simulink model "ejemplo_mimo"  (R2018a)
settings: Solver=VariableStepAuto  StartTime=0.0  StopTime=10  RelTol=1e-3
InitFcn:
  | ej_mimo2
values from neighbouring files (symbols this model uses):
  ki = kt(1,3)    [control_nolineal_linealizacion_entrada_estado.m]    (also in e_mimo.m; ej_mimo.m = kt(:,2+1:end); ej_mimo2.m = kt(:,2+1:end); ejemplo_2.m)
  kp = kt(1,1:2)    [control_nolineal_linealizacion_entrada_estado.m]    (also in e_mimo.m; ej_mimo.m = kt(:,1:2); ej_mimo2.m = kt(:,1:2); ejemplo_2.m)
libraries: simulink x2
settings Model: Creator=carma  LastModifiedBy=carma

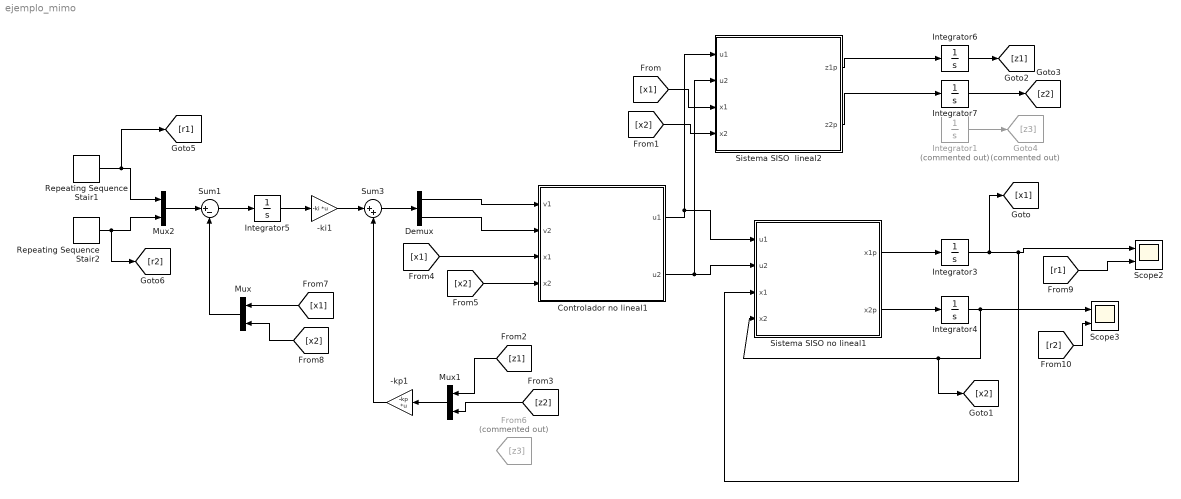
== system ejemplo_mimo ==
  -ki1 : Gain  Gain=-ki  Multiplication=Matrix(K*u) (u vector)
  -kp1 : Gain  Gain=-kp  Multiplication=Matrix(K*u) (u vector)
  Controlador no lineal1 : MATLAB Function  TreatAsAtomicUnit=on
  Demux : Demux  Outputs=2
  From6 : From  Commented=on  GotoTag=z3
  Goto4 : Goto  Commented=on  GotoTag=z3
  Integrator1 : Integrator  Commented=on
  Integrator{3..7} (5 alike) : Integrator
  Mux : Mux  Inputs=2
  Mux1 : Mux  Inputs=2
  Mux2 : Mux  Inputs=2
  Repeating Sequence Stair1 : simulink/Sources/Repeating Sequence Stair  OutValues=[0.5 0.4 -0.2 0.1 0.3].'  tsamp=2  OutMin=[]  OutMax=[]  OutDataTypeStr=double  OutputDataTypeScalingMode=double  OutDataType=fixdt(0,8)  ConRadixGroup=Best Precision: Vector-wise  OutScaling=2^-12
  Repeating Sequence Stair2 : simulink/Sources/Repeating Sequence Stair  OutValues=[-0.5 -0.4 0.2 -0.1 -0.3].'  tsamp=1.5  OutMin=[]  OutMax=[]  OutDataTypeStr=double  OutputDataTypeScalingMode=double  OutDataType=fixdt(0,8)  ConRadixGroup=Best Precision: Vector-wise  OutScaling=2^-12
  Scope2 : Scope  NumInputPorts=2
  Scope3 : Scope  NumInputPorts=2
  Sistema SISO  lineal2 : MATLAB Function  TreatAsAtomicUnit=on
  Sistema SISO no lineal1 : MATLAB Function  TreatAsAtomicUnit=on
  Sum1 : Sum  Inputs=|+-
  Sum3 : Sum  Inputs=|++
  wires:
  Sistema SISO  lineal2/1(z1p) -> Integrator6/1
  Sistema SISO no lineal1/2(x2p) -> Integrator4/1
  Sum1/1 -> Integrator5/1
  Controlador no lineal1/1(u1) -> Sistema SISO no lineal1/1(u1), Sistema SISO  lineal2/1(u1)
  Sistema SISO no lineal1/1(x1p) -> Integrator3/1
  Integrator4/1 -> [x2], Sistema SISO no lineal1/4(x2), Scope3/1
  Mux1/1 -> -kp1/1
  Integrator5/1 -> -ki1/1
  Sistema SISO  lineal2/2(z2p) -> Integrator7/1
  -ki1/1 -> Sum3/1
  -kp1/1 -> Sum3/2
  Integrator3/1 -> [x1], Scope2/1, Sistema SISO no lineal1/3(x1)
  [x1] -> Sistema SISO  lineal2/3(x1)
  [x2] -> Sistema SISO  lineal2/4(x2)
  Integrator6/1 -> [z1]
  Integrator7/1 -> [z2]
  [z1] -> Mux1/1
  [z2] -> Mux1/2
  Integrator1/1 -> Goto4/1
  Mux2/1 -> Sum1/1
  Repeating Sequence Stair1/1 -> [r1], Mux2/1
  Repeating Sequence Stair2/1 -> [r2], Mux2/2
  [x1] -> Mux/1
  [x2] -> Mux/2
  Mux/1 -> Sum1/2
  [r1] -> Scope2/2
  [r2] -> Scope3/2
  Sum3/1 -> Demux/1
  Demux/1 -> Controlador no lineal1/1(v1)
  [x2] -> Controlador no lineal1/4(x2)
  [x1] -> Controlador no lineal1/3(x1)
  Demux/2 -> Controlador no lineal1/2(v2)
  Controlador no lineal1/2(u2) -> Sistema SISO  lineal2/2(u2), Sistema SISO no lineal1/2(u2)

== matlab function ejemplo_mimo/Controlador no lineal1 ==
  data: v1 input; u1 output; v2 input; x1 input; x2 input; u2 output
function [u1,u2] = fcn(v1,v2,x1,x2)

%parametros



% u=0.5*(v1-2*x1^2-3*x1^2*(x1^3+x2)+v2);
u1=v1-x1^3-x2;
u2=v2-x1^2;

% u=v1-x1^2-3*x1^2*(x1^3+x2);

% u=v2-x1^2;
%s=5;
%syms y
%Cx3=(2+10^(pk2-y))/(1+10^(pk2-y)+10^(pk1+pk2-2*y));
%h=-x1+x2-x3*Cx3+10^(-y)-10^(y-pkw)==0;

%s=double(solve(h));

== matlab function ejemplo_mimo/Sistema SISO no lineal1 ==
  data: u1 input; u2 input; x1p output; x1 input; x2 input; x2p output
function [x1p,x2p]= fcn(u1,u2,x1,x2)

%parametros
a=4;



x1p=x2+x1^3+u1;
x2p=x1^2+u2;

%s=5;
%syms y
%Cx3=(2+10^(pk2-y))/(1+10^(pk2-y)+10^(pk1+pk2-2*y));
%h=-x1+x2-x3*Cx3+10^(-y)-10^(y-pkw)==0;

%s=double(solve(h));

== matlab function ejemplo_mimo/Sistema SISO  lineal2 ==
  data: u1 input; u2 input; z1p output; x1 input; x2 input; z2p output
function [z1p,z2p]= fcn(u1,u2,x1,x2)

z1p=x1^3+x2+u1;
z2p=x1^2+u2;


% z1p=x2+x1^3;
% z2p=x1^2+u;
% z3p=u+x1^2+3*x1^2*(x2+x1^3);


% z1p=z2;
% z2p=v;

%s=5;
%syms y
%Cx3=(2+10^(pk2-y))/(1+10^(pk2-y)+10^(pk1+pk2-2*y));
%h=-x1+x2-x3*Cx3+10^(-y)-10^(y-pkw)==0;

%s=double(solve(h));
